simulink model "ROS_Controller"  (R2015b)
settings: Solver=ode3  StartTime=0.0  StopTime=inf  FixedStep=0.05  RelTol=1e-3
undefined symbols (not defined in the file): C_nuParams, D, D_nuParams, InitialPos, invM, invT, invThrustAloc, K2, K3, K4, Kd, Ki, Kp, Sat1Low, Sat1Up, Sat2Low, Sat2Up, Tr, wni, wniCeta2, wnisquared, X, Y, Z
libraries: robotlib x4, realtime_pacer_lib x1
settings Model: Creator=einar  LastModifiedBy=einar
settings DataIOCC: ReturnWorkspaceOutputs=on
settings OptimizationCC: OptimizeModelRefInitCode=on  LifeSpan=Inf  MaxStackSize=64
settings DebuggingCC: ReadBeforeWriteMsg=DisableAll  WriteAfterWriteMsg=DisableAll  WriteAfterReadMsg=DisableAll  MultiTaskDSMMsg=none
settings HardwareCC: ProdBitPerPointer=32  ProdLargestAtomicFloat=None  ProdIntDivRoundTo=Undefined  ProdEndianess=Unspecified  ProdWordSize=32  ProdHWDeviceType=Generic->Unspecified (assume 32-bit Generic)
settings ModelReferenceCC: UpdateModelReferenceTargets=IfOutOfDate
settings SFSimCC: SFSimEcho=off
settings RTWCC: SystemTargetFile=ert.tlc  TemplateMakefile=ert_default_tmf  Description=Embedded Coder  Toolchain=Catkin  TargetLang=C++
settings CodeAppCC: IgnoreCustomStorageClasses=off
settings ERTTargetCC: SupportContinuousTime=on

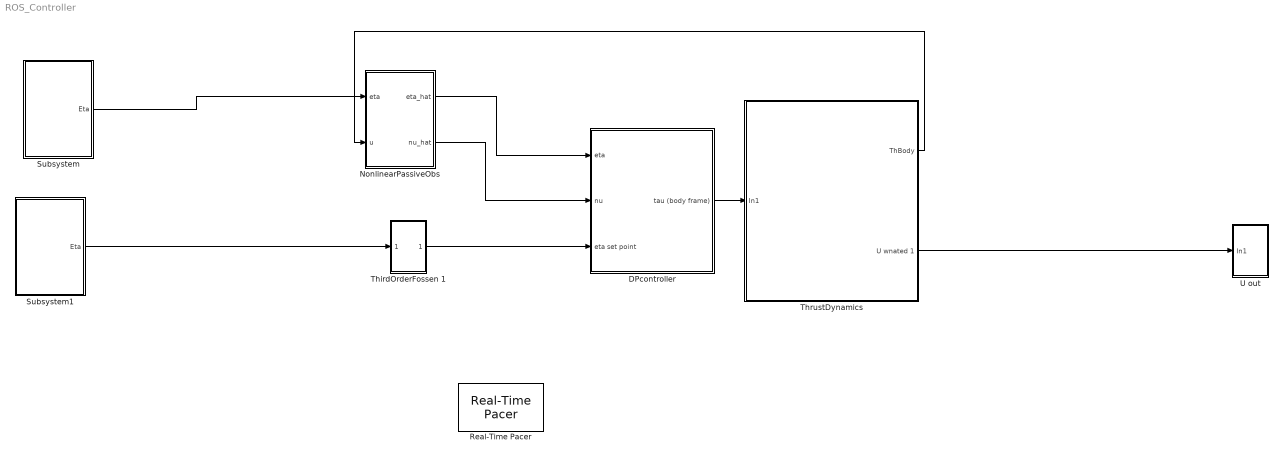
== system ROS_Controller ==
  DPcontroller : Subsystem
  NonlinearPassiveObs : Subsystem
  Real-Time Pacer : realtime_pacer_lib/Real-Time Pacer  simTimePerRealTime=1
  Subsystem : Subsystem
  Subsystem1 : Subsystem
  ThirdOrderFossen 1 : Subsystem
  ThrustDynamics : Subsystem
  U out : Subsystem
  wires:
  ThrustDynamics/2(U wnated 1) -> U out/1(In1)
  NonlinearPassiveObs/1(eta_hat) -> DPcontroller/1(eta)
  NonlinearPassiveObs/2(nu_hat) -> DPcontroller/2(nu)
  DPcontroller/1(tau (body frame)) -> ThrustDynamics/1(In1)
  ThrustDynamics/1("ThBody ") -> NonlinearPassiveObs/2(u)
  ThirdOrderFossen 1/1(Out1) -> DPcontroller/3(eta set point)
  Subsystem/1(Eta) -> NonlinearPassiveObs/1(eta)
  Subsystem1/1(Eta) -> ThirdOrderFossen 1/1(In1)

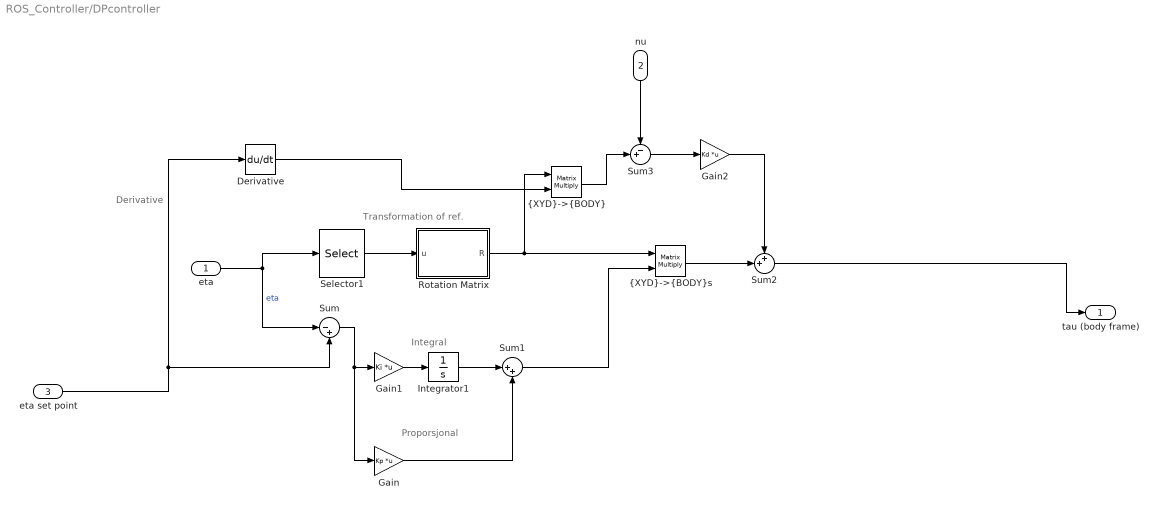
== system ROS_Controller/DPcontroller ==
  note: Integral
  note: Proporsjonal
  note: Transformation of ref.
  note: Derivative
  eta : Inport
  nu : Inport  Port=2
  eta set point : Inport  Port=3
  Derivative : Derivative
  Gain : Gain  Gain=Kp  Multiplication=Matrix(K*u)
  Gain1 : Gain  Gain=Ki  Multiplication=Matrix(K*u)
  Gain2 : Gain  Gain=Kd  Multiplication=Matrix(K*u)
  Integrator1 : Integrator  InitialCondition=[0;0;0]  LimitOutput=on  UpperSaturationLimit=[1;1;1]  LowerSaturationLimit=[-1;-1;-1]
  Rotation Matrix : MATLAB Function  TreatAsAtomicUnit=on
  Selector1 : Selector  InputPortWidth=3  IndexOptions=Index vector (dialog)  Indices=[3]  OutputSizes=1
  Sum : Sum  Inputs=|-+
  Sum1 : Sum  Inputs=|++
  Sum2 : Sum  Inputs=++|
  Sum3 : Sum  Inputs=-+|
  "{XYD}->{BODY}" : Product  Multiplication=Matrix(*)
  "{XYD}->{BODY}s" : Product  Multiplication=Matrix(*)
  tau (body frame) : Outport
  wires:
  eta/1 -> Selector1/1, Sum/1  "eta"
  Sum/1 -> Gain1/1, Gain/1
  Selector1/1 -> Rotation Matrix/1(u)
  Rotation Matrix/1(R) -> "{XYD}->{BODY}"/1, "{XYD}->{BODY}s"/1
  Sum2/1 -> tau (body frame)/1
  Gain1/1 -> Integrator1/1
  Gain/1 -> Sum1/2
  Sum1/1 -> "{XYD}->{BODY}s"/2
  Derivative/1 -> "{XYD}->{BODY}"/2
  "{XYD}->{BODY}s"/1 -> Sum2/2
  nu/1 -> Sum3/1
  "{XYD}->{BODY}"/1 -> Sum3/2
  Sum3/1 -> Gain2/1
  Gain2/1 -> Sum2/1
  eta set point/1 -> Sum/2, Derivative/1
  Integrator1/1 -> Sum1/1

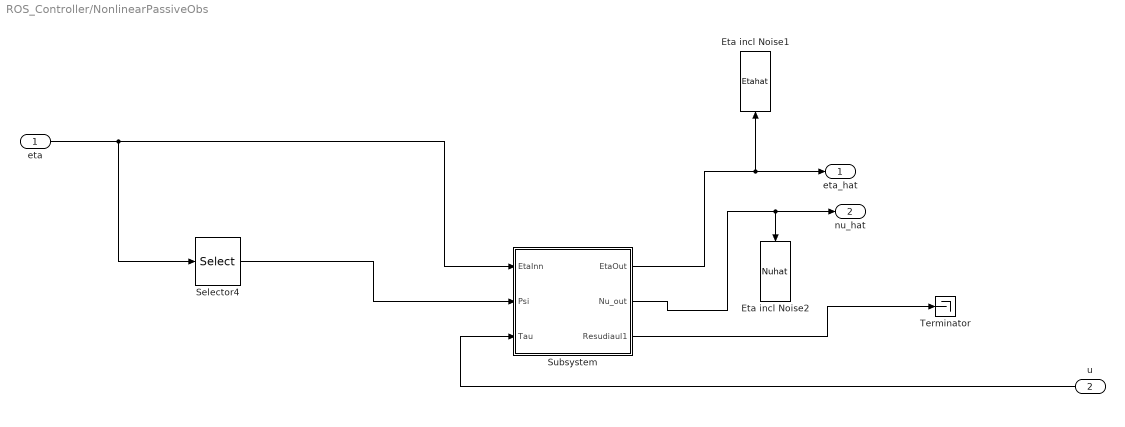
== system ROS_Controller/NonlinearPassiveObs ==
  eta : Inport
  u : Inport  Port=2
  Eta incl Noise1 : ToWorkspace  VariableName=Etahat  SaveFormat=Timeseries  SampleTime=-1
  Eta incl Noise2 : ToWorkspace  VariableName=Nuhat  SaveFormat=Timeseries  SampleTime=-1
  Selector4 : Selector  InputPortWidth=3  IndexOptions=Index vector (dialog)  Indices=3  OutputSizes=1
  Subsystem : Subsystem
  Terminator : Terminator
  eta_hat : Outport
  nu_hat : Outport  Port=2
  wires:
  Subsystem/3("Resudiaul1 ") -> Terminator/1
  eta/1 -> Selector4/1, Subsystem/1(EtaInn)
  Selector4/1 -> Subsystem/2(Psi)
  u/1 -> Subsystem/3("Tau ")
  Subsystem/2("Nu_out ") -> Eta incl Noise2/1, nu_hat/1
  Subsystem/1("EtaOut ") -> Eta incl Noise1/1, eta_hat/1

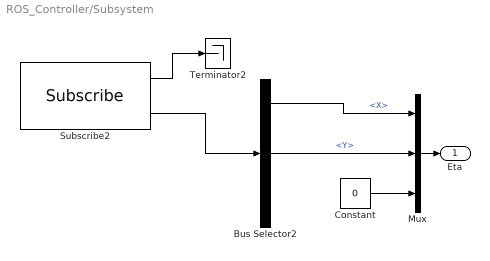
== system ROS_Controller/Subsystem ==
  Bus Selector2 : BusSelector  OutputSignals=X,Y,Z
  Constant : Constant  Value=0
  Mux : Mux  Inputs=3
  Subscribe2 : robotlib/Subscribe  SourceLibraryInfo=This block requires Robotics System Toolbox  topicSource=Specify your own  topic=/Eta  messageType=geometry_msgs/Vector3  sampleTime=-1  messageQueueLength=1
  Terminator2 : Terminator
  Eta : Outport
  wires:
  Bus Selector2/1 -> Mux/1  "<X>"
  Subscribe2/2 -> Bus Selector2/1
  Mux/1 -> Eta/1
  Subscribe2/1 -> Terminator2/1
  Bus Selector2/2 -> Mux/2  "<Y>"
  Constant/1 -> Mux/3

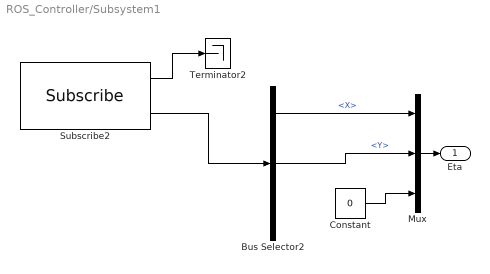
== system ROS_Controller/Subsystem1 ==
  Bus Selector2 : BusSelector  OutputSignals=X,Y,Z
  Constant : Constant  Value=0
  Mux : Mux  Inputs=3
  Subscribe2 : robotlib/Subscribe  SourceLibraryInfo=This block requires Robotics System Toolbox  topicSource=Specify your own  topic=/EtaSet  messageType=geometry_msgs/Vector3  sampleTime=-1  messageQueueLength=1
  Terminator2 : Terminator
  Eta : Outport
  wires:
  Subscribe2/2 -> Bus Selector2/1
  Mux/1 -> Eta/1
  Subscribe2/1 -> Terminator2/1
  Bus Selector2/1 -> Mux/1  "<X>"
  Bus Selector2/2 -> Mux/2  "<Y>"
  Constant/1 -> Mux/3

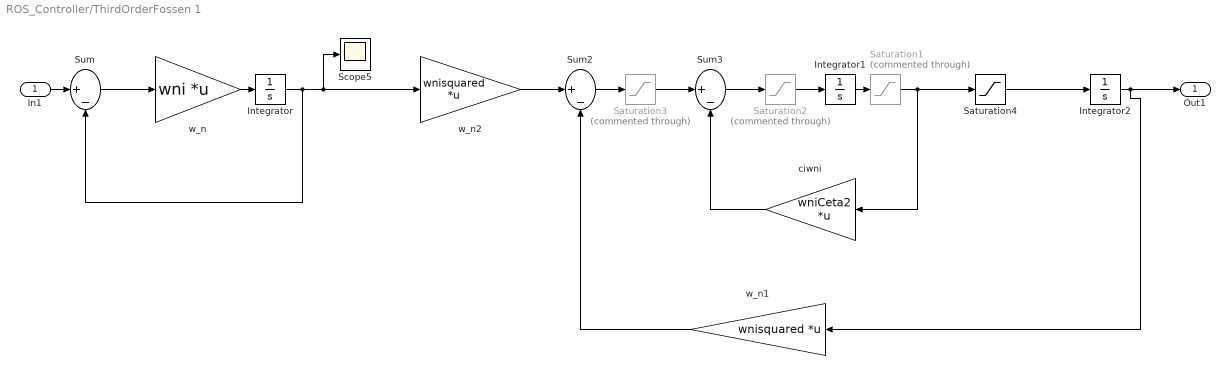
== system ROS_Controller/ThirdOrderFossen 1 ==
  In1 : Inport
  Integrator : Integrator  InitialCondition=[0;0;0]
  Integrator1 : Integrator  InitialCondition=[0 ;0; 0]
  Integrator2 : Integrator  InitialCondition=[0;0;0]
  Saturation1 : Saturate  Commented=through  UpperLimit=Sat2Up  LowerLimit=Sat2Low
  Saturation2 : Saturate  Commented=through  UpperLimit=Sat1Up  LowerLimit=Sat1Low
  Saturation3 : Saturate  Commented=through  UpperLimit=Sat1Up  LowerLimit=Sat1Low
  Saturation4 : Saturate  UpperLimit=Sat2Up  LowerLimit=Sat2Low
  Scope5 : Scope
  Sum : Sum  Inputs=|+-
  Sum2 : Sum  Inputs=|+-
  Sum3 : Sum  Inputs=|+-
  ciwni : Gain  Gain=wniCeta2  Multiplication=Matrix(K*u)
  w_n : Gain  Gain=wni  Multiplication=Matrix(K*u)
  w_n1 : Gain  Gain=wnisquared  Multiplication=Matrix(K*u)
  w_n2 : Gain  Gain=wnisquared  Multiplication=Matrix(K*u)
  Out1 : Outport
  wires:
  w_n/1 -> Integrator/1
  w_n2/1 -> Sum2/1
  Integrator/1 -> Scope5/1, w_n2/1, Sum/2
  Integrator2/1 -> Out1/1, w_n1/1
  ciwni/1 -> Sum3/2
  Saturation1/1 -> ciwni/1, Saturation4/1
  Saturation2/1 -> Integrator1/1
  Sum2/1 -> Saturation3/1
  Sum3/1 -> Saturation2/1
  Sum/1 -> w_n/1
  In1/1 -> Sum/1
  Integrator1/1 -> Saturation1/1
  w_n1/1 -> Sum2/2
  Saturation3/1 -> Sum3/1
  Saturation4/1 -> Integrator2/1

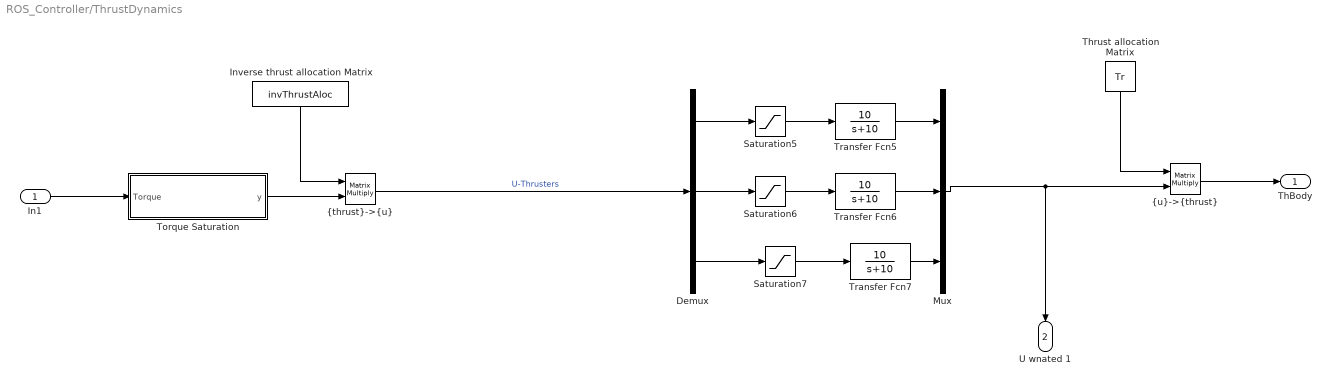
== system ROS_Controller/ThrustDynamics ==
  In1 : Inport
  Demux : Demux  Outputs=3
  Inverse thrust allocation Matrix : Constant  Value=invThrustAloc
  Mux : Mux  Inputs=3
  Saturation5 : Saturate  UpperLimit=4  LowerLimit=-4  ZeroCross=off
  Saturation6 : Saturate  UpperLimit=4  LowerLimit=-4  ZeroCross=off
  Saturation7 : Saturate  UpperLimit=4  LowerLimit=-4  ZeroCross=off
  Thrust allocation Matrix : Constant  Value=Tr
  Torque Saturation : MATLAB Function  TreatAsAtomicUnit=on
  Transfer Fcn5 : TransferFcn  Numerator=[10]  Denominator=[1 10]
  Transfer Fcn6 : TransferFcn  Numerator=[10]  Denominator=[1 10]
  Transfer Fcn7 : TransferFcn  Numerator=[10]  Denominator=[1 10]
  "{thrust}->{u}" : Product  Multiplication=Matrix(*)
  "{u}->{thrust}" : Product  Multiplication=Matrix(*)
  "ThBody " : Outport
  U wnated 1 : Outport  Port=2
  wires:
  Demux/1 -> Saturation5/1
  Demux/2 -> Saturation6/1
  Demux/3 -> Saturation7/1
  "{u}->{thrust}"/1 -> "ThBody "/1
  Thrust allocation Matrix/1 -> "{u}->{thrust}"/1
  Mux/1 -> U wnated 1/1, "{u}->{thrust}"/2
  "{thrust}->{u}"/1 -> Demux/1  "U-Thrusters"
  Inverse thrust allocation Matrix/1 -> "{thrust}->{u}"/1
  In1/1 -> Torque Saturation/1(Torque)
  Torque Saturation/1(y) -> "{thrust}->{u}"/2
  Saturation7/1 -> Transfer Fcn7/1
  Saturation6/1 -> Transfer Fcn6/1
  Saturation5/1 -> Transfer Fcn5/1
  Transfer Fcn5/1 -> Mux/1
  Transfer Fcn7/1 -> Mux/3
  Transfer Fcn6/1 -> Mux/2

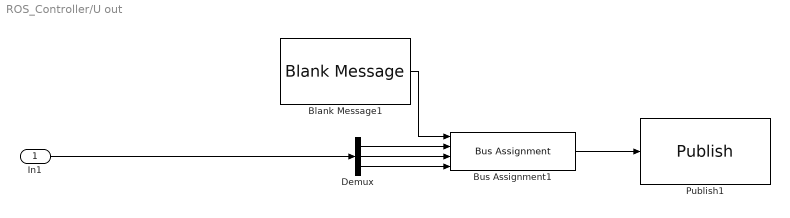
== system ROS_Controller/U out ==
  In1 : Inport
  Blank Message1 : robotlib/Blank Message  SourceLibraryInfo=This block requires Robotics System Toolbox  messageType=geometry_msgs/Vector3  SampleTime=inf
  Bus Assignment1 : BusAssignment  AssignedSignals=X,Y,Z
  Demux : Demux  Outputs=3
  Publish1 : robotlib/Publish  SourceLibraryInfo=This block requires Robotics System Toolbox  topicSource=Specify your own  topic=/U  messageType=geometry_msgs/Vector3  messageQueueLength=1
  wires:
  Bus Assignment1/1 -> Publish1/1
  Blank Message1/1 -> Bus Assignment1/1
  In1/1 -> Demux/1
  Demux/1 -> Bus Assignment1/2
  Demux/2 -> Bus Assignment1/3
  Demux/3 -> Bus Assignment1/4

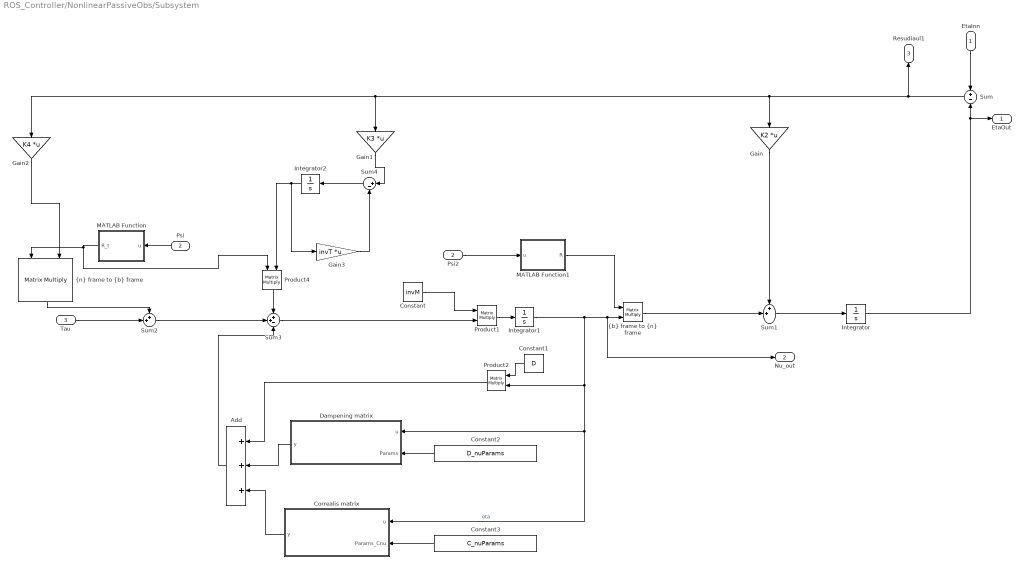
== system ROS_Controller/NonlinearPassiveObs/Subsystem ==
  EtaInn : Inport
  Psi : Inport  Port=2
  "Tau " : Inport  Port=3
  Add : Sum  Inputs=+++
  Constant : Constant  Value=invM
  Constant1 : Constant  Value=D
  Constant2 : Constant  Value=D_nuParams
  Constant3 : Constant  Value=C_nuParams
  Correalis matrix : MATLAB Function  TreatAsAtomicUnit=on
  Dampening matrix : MATLAB Function  TreatAsAtomicUnit=on
  Gain : Gain  Gain=K2  Multiplication=Matrix(K*u)
  Gain1 : Gain  Gain=K3  Multiplication=Matrix(K*u)
  Gain2 : Gain  Gain=K4  Multiplication=Matrix(K*u)
  Gain3 : Gain  Gain=invT  Multiplication=Matrix(K*u)
  Integrator : Integrator  InitialCondition=InitialPos
  Integrator1 : Integrator
  Integrator2 : Integrator  InitialCondition=[0;0;0]
  MATLAB Function : MATLAB Function  TreatAsAtomicUnit=on
  MATLAB Function1 : MATLAB Function  TreatAsAtomicUnit=on
  Product1 : Product  Multiplication=Matrix(*)
  Product2 : Product  Multiplication=Matrix(*)
  Product4 : Product  Multiplication=Matrix(*)
  Psi2 : InportShadow  Port=2
  Sum : Sum  Inputs=+|-
  Sum1 : Sum  Inputs=++|
  Sum2 : Sum  Inputs=++|
  Sum3 : Sum  Inputs=++-
  Sum4 : Sum  Inputs=|+-
  "{b} frame to {n} frame" : Product  Multiplication=Matrix(*)
  "{n} frame to {b} frame" : Product  Multiplication=Matrix(*)
  "EtaOut " : Outport
  "Nu_out " : Outport  Port=2
  "Resudiaul1 " : Outport  Port=3
  wires:
  Add/1 -> Sum3/3
  Correalis matrix/1(y) -> Add/3
  Dampening matrix/1(y) -> Add/2
  Product2/1 -> Add/1
  Integrator1/1 -> Product2/2, Dampening matrix/1(u), Correalis matrix/1(u), "Nu_out "/1, "{b} frame to {n} frame"/2  "eta"
  Constant3/1 -> Correalis matrix/2(Params_Cnu)
  Constant2/1 -> Dampening matrix/2(Params)
  Gain2/1 -> "{n} frame to {b} frame"/2
  EtaInn/1 -> Sum/1
  Sum/1 -> "Resudiaul1 "/1, Gain2/1, Gain1/1, Gain/1
  Gain/1 -> Sum1/1
  Sum1/1 -> Integrator/1
  Integrator/1 -> Sum/2, "EtaOut "/1
  Psi/1 -> MATLAB Function/1(u)
  "{n} frame to {b} frame"/1 -> Sum2/1
  "Tau "/1 -> Sum2/2
  Constant/1 -> Product1/1
  Product1/1 -> Integrator1/1
  Constant1/1 -> Product2/1
  Sum2/1 -> Sum3/2
  Sum3/1 -> Product1/2
  Psi2/1 -> MATLAB Function1/1(u)
  MATLAB Function1/1(R) -> "{b} frame to {n} frame"/1
  MATLAB Function/1(R_t) -> Product4/1, "{n} frame to {b} frame"/1
  "{b} frame to {n} frame"/1 -> Sum1/2
  Gain1/1 -> Sum4/1
  Sum4/1 -> Integrator2/1
  Integrator2/1 -> Product4/2, Gain3/1
  Gain3/1 -> Sum4/2
  Product4/1 -> Sum3/1

== matlab function ROS_Controller/DPcontroller/Rotation Matrix ==
  data: u input; R output
function R = fcn(u)
RotPhi=[cos(u) -sin(u) 0;sin(u) cos(u) 0 ;0 0 1];
R = RotPhi';
%R=[RotPhi(1:2,:);[0 0 0;0 0 0;0 0 0];RotPhi(3,:)]
end

== matlab function ROS_Controller/NonlinearPassiveObs/Subsystem/Correalis matrix ==
  data: u input; y output; Params_Cnu input
function y = fcn(u,Params_Cnu)
%#codegen
C=[0 Params_Cnu(2,1)*u(3) 0;-Params_Cnu(1,2)*u(3) 0 0;0 0 0];
y=C*u;

== matlab function ROS_Controller/NonlinearPassiveObs/Subsystem/Dampening matrix ==
  data: u input; y output; Params input
function y = fcn(u,Params)
%#codegen
Dnu=[Params(1,1)*abs(u(1)) 0 0;0 Params(2,2)*abs(u(2)) 0;0 0 0];
y=Dnu*u;

== matlab function ROS_Controller/NonlinearPassiveObs/Subsystem/MATLAB Function ==
  data: u input; R_t output
function R_t = fcn(u)
RotPhi=[cos(u) -sin(u) 0;sin(u) cos(u) 0 ;0 0 1];
R_t = RotPhi';
%R=[RotPhi(1:2,:);[0 0 0;0 0 0;0 0 0];RotPhi(3,:)]
end

== matlab function ROS_Controller/NonlinearPassiveObs/Subsystem/MATLAB Function1 ==
  data: u input; R output
function R = fcn(u)
RotPhi=[cos(u) -sin(u) 0;sin(u) cos(u) 0 ;0 0 1];
R = RotPhi;
end

== matlab function ROS_Controller/ThrustDynamics/Torque Saturation ==
  data: Torque input; y output
function y = fcn(Torque)
F_max=3.7;
Com_Torque=norm(Torque(1:2));
if Com_Torque>F_max
Torque(1:2,1)=Torque(1:2,1).*(F_max/Com_Torque)    ;
end
T_max=0.3;
if abs(Torque(3))>T_max
Torque(3)=T_max*Torque(3)/abs(Torque(3));
end;
y=Torque;
